simulink model "SoftRoboticTentacle"  (R2024b)
settings: Solver=FixedStepAuto  StartTime=0.0  StopTime=0.1  FixedStep=0.01  RelTol=1e-3
undefined symbols (not defined in the file): c, k, m
settings Model: Creator=Robin  LastModifiedBy=Robin
settings RTWCC: GPUComputeCapability=3.5

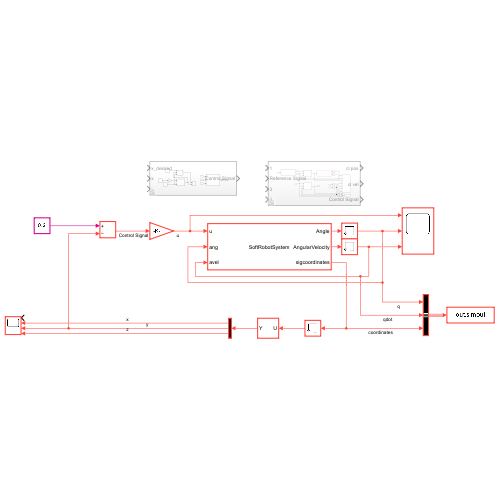
[thumbnail: Simulink's stored preview of the top-level diagram]
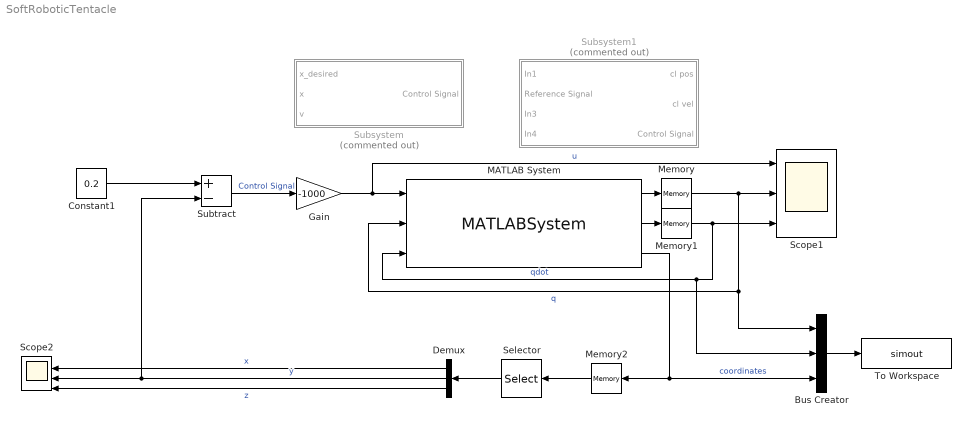
== system SoftRoboticTentacle ==
  Bus Creator : BusCreator  Inputs=3
  Constant1 : Constant  Value=0.2
  Demux : Demux  Outputs=3
  Gain : Gain  Gain=-1000
  MATLAB System : MATLABSystem  System=SoftRobotSystem  SimulateUsing=Interpreted execution
      mask Type: SoftRobotSystem
      mask Display:
      | disp('SoftRobotSystem');
      | port_label('input',1,'u');
      | port_label('input',2,'ang');
      | port_label('input',3,'avel');
      | port_label('output',1,'Angle');
      | port_label('output',2,'AngularVelocity');
      | port_label('output',3,'sigcoordinates');
  Memory : Memory
  Memory1 : Memory
  Memory2 : Memory
  Scope1 : Scope  NumInputPorts=3
  Scope2 : Scope  NumInputPorts=4
  Selector : Selector  InputPortWidth=24  IndexOptions=Index vector (dialog)  Indices=[22 23 24]  OutputSizes=1
  Subsystem : Subsystem  Commented=on
  Subsystem1 : Subsystem  Commented=on
  Subtract : Sum  Inputs=+-
  To Workspace : ToWorkspace  VariableName=simout  SaveFormat=Timeseries  SampleTime=-1
  wires:
  MATLAB System/2 -> Memory1/1
  Bus Creator/1 -> To Workspace/1
  Memory/1 -> Scope1/2, Bus Creator/1, MATLAB System/2  "q"
  Memory1/1 -> Scope1/3, Bus Creator/2, MATLAB System/3  "qdot"
  MATLAB System/1 -> Memory/1
  MATLAB System/3 -> Memory2/1, Bus Creator/3  "coordinates"
  Selector/1 -> Demux/1
  Demux/2 -> Subtract/2, Scope2/3  "y"
  Demux/1 -> Scope2/2  "x"
  Demux/3 -> Scope2/4  "z"
  Constant1/1 -> Subtract/1
  Subtract/1 -> Gain/1  "Control Signal"
  Gain/1 -> Scope1/1, MATLAB System/1  "u"
  Memory2/1 -> Selector/1

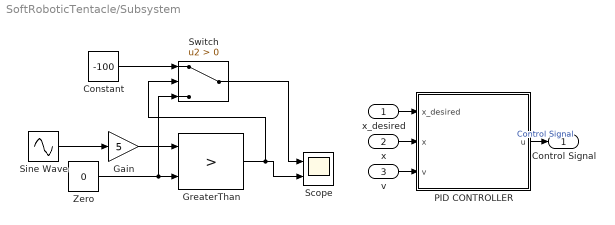
== system SoftRoboticTentacle/Subsystem ==
  x_desired : Inport
  x : Inport  Port=2
  v : Inport  Port=3
  Constant : Constant  Value=-100
  Gain : Gain  Gain=5
  GreaterThan : RelationalOperator  Operator=>  OutDataTypeStr=boolean  RndMeth=Simplest  InputSameDT=off
  PID CONTROLLER : MATLAB Function  TreatAsAtomicUnit=on
  Scope : Scope  NumInputPorts=2
  Sine Wave : Sin  Frequency=10  SampleTime=0
  Switch : Switch  Criteria=u2 > Threshold  SaturateOnIntegerOverflow=off  InputSameDT=off
  Zero : Constant  Value=0  OutDataTypeStr=Inherit: Inherit via back propagation
  Control Signal : Outport
  wires:
  Gain/1 -> GreaterThan/1
  Switch/1 -> Scope/1
  GreaterThan/1 -> Switch/2, Scope/2
  Zero/1 -> Switch/3, GreaterThan/2
  Sine Wave/1 -> Gain/1
  Constant/1 -> Switch/1
  x/1 -> PID CONTROLLER/2(x)
  v/1 -> PID CONTROLLER/3(v)
  x_desired/1 -> PID CONTROLLER/1(x_desired)
  PID CONTROLLER/1(u) -> Control Signal/1  "Control Signal"

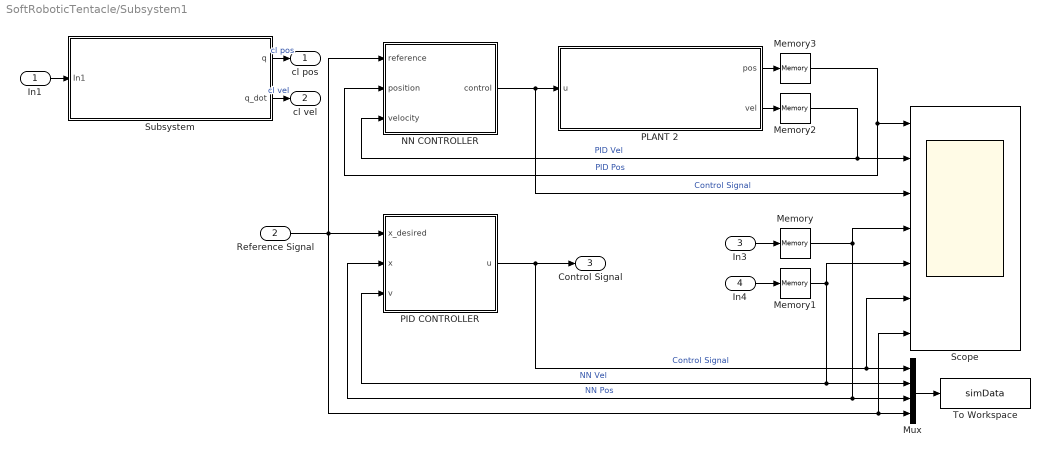
== system SoftRoboticTentacle/Subsystem1 ==
  In1 : Inport
  Reference Signal : Inport  Port=2
  In3 : Inport  Port=3
  In4 : Inport  Port=4
  Memory{,1..3} (4 alike) : Memory
  Mux : Mux
  NN CONTROLLER : MATLAB Function  TreatAsAtomicUnit=on
  PID CONTROLLER : MATLAB Function  TreatAsAtomicUnit=on
  PLANT 2 : MATLAB Function  TreatAsAtomicUnit=on  SystemSampleTime=0.01
  Scope : Scope  NumInputPorts=7
  Subsystem : Subsystem
  To Workspace : ToWorkspace  VariableName=simData  SaveFormat=Structure With Time  SampleTime=-1
  cl pos : Outport
  cl vel : Outport  Port=2
  Control Signal : Outport  Port=3
  wires:
  Memory2/1 -> NN CONTROLLER/3(velocity), Scope/2  "PID Vel"
  Memory/1 -> Scope/4, PID CONTROLLER/2(x), Mux/3  "NN Pos"
  PLANT 2/1(pos) -> Memory3/1
  Memory1/1 -> Scope/5, PID CONTROLLER/3(v), Mux/2  "NN Vel"
  Mux/1 -> To Workspace/1
  PID CONTROLLER/1(u) -> Control Signal/1, Mux/1, Scope/6  "Control Signal"
  NN CONTROLLER/1(control) -> Scope/3, PLANT 2/1(u)  "Control Signal"
  Reference Signal/1 -> PID CONTROLLER/1(x_desired), NN CONTROLLER/1(reference), Scope/7, Mux/4
  Memory3/1 -> NN CONTROLLER/2(position), Scope/1  "PID Pos"
  PLANT 2/2(vel) -> Memory2/1
  In1/1 -> Subsystem/1(In1)
  Subsystem/1(q) -> cl pos/1  "cl pos"
  Subsystem/2(q_dot) -> cl vel/1  "cl vel"
  In4/1 -> Memory1/1
  In3/1 -> Memory/1

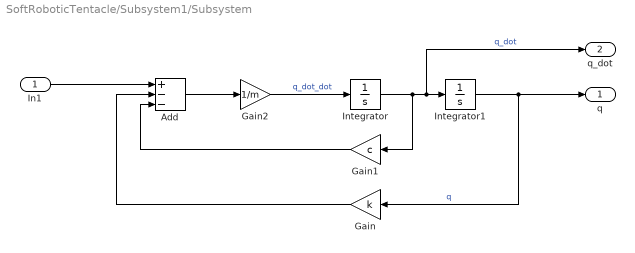
== system SoftRoboticTentacle/Subsystem1/Subsystem ==
  In1 : Inport
  Add : Sum  Inputs=+--
  Gain : Gain  Gain=k
  Gain1 : Gain  Gain=c
  Gain2 : Gain  Gain=1/m
  Integrator : Integrator
  Integrator1 : Integrator
  q : Outport
  q_dot : Outport  Port=2
  wires:
  Gain/1 -> Add/2
  Gain2/1 -> Integrator/1  "q_dot_dot"
  Integrator1/1 -> q/1, Gain/1  "q"
  Gain1/1 -> Add/3
  Integrator/1 -> Gain1/1, q_dot/1, Integrator1/1  "q_dot"
  Add/1 -> Gain2/1
  In1/1 -> Add/1

== matlab function SoftRoboticTentacle/Subsystem1/PID CONTROLLER ==
  settings: updateMethod=DISCRETE
  data: x_desired input; u output; x input; v input
function u = PIDController(x_desired, x, v)
% PIDController - Classic PID controller for mass-spring-damper system
%
% Inputs:
%   x_desired - Desired position (reference)
%   x         - Current position
%   v         - Current velocity
%
% Output:
%   u         - Control force

% Controller gains
Kp = 10;
Ki = 2;
Kd = 2;

% Sample time
Ts = 0.01;

% Persistent PID states
persistent integral_error prev_error
if isempty(integral_error)
    integral_error = 0;
    prev_error = 0;
end

% Compute errors
position_error = x_desired - x;
integral_error = integral_error + position_error * Ts;
derivative_error = (position_error - prev_error) / Ts;

% PID control law
u = Kp * position_error + Ki * integral_error + Kd * derivative_error;

% Optional: Saturation
% u = max(min(u, 10), -10);

% Update persistent state
prev_error = position_error;
end

== matlab function SoftRoboticTentacle/Subsystem/PID CONTROLLER ==
  settings: updateMethod=DISCRETE
  data: x_desired input; u output; x input; v input
function u = PIDController(x_desired, x, v)
% PIDController - Classic PID controller for mass-spring-damper system
%
% Inputs:
%   x_desired - Desired position (reference)
%   x         - Current position
%   v         - Current velocity
%
% Output:
%   u         - Control force

% Controller gains
Kp = 10;
Ki = 2;
Kd = 2;

% Sample time
Ts = 0.01;

% Persistent PID states
persistent integral_error prev_error
if isempty(integral_error)
    integral_error = 0;
    prev_error = 0;
end

% Compute errors
position_error = x_desired - x;
integral_error = integral_error + position_error * Ts;
derivative_error = (position_error - prev_error) / Ts;

% PID control law
u = Kp * position_error + Ki * integral_error + Kd * derivative_error;

% Optional: Saturation
% u = max(min(u, 10), -10);

% Update persistent state
prev_error = position_error;
end

== matlab function SoftRoboticTentacle/Subsystem1/NN CONTROLLER ==
  data: reference input; control output; position input; velocity input
function control = NN_controller(reference, position, velocity)

input = [reference; position; velocity];

control = NNController(input);

== matlab function SoftRoboticTentacle/Subsystem1/PLANT 2 ==
  data: u input; pos output; vel output
function [pos, vel] = massSpringDamperDynamics(u)
% Discrete-time mass-spring-damper system
% u: input force (N)
% pos: output position (m)
% vel: output velocity (m/s)

% System parameters
m = 1.0;    % Mass (kg)
c = 0.5;    % Damping coefficient (Ns/m)
k = 2.0;    % Spring constant (N/m)
Ts = 0.01;  % Sample time (s)

% Persistent state variables
persistent x_prev v_prev
if isempty(x_prev)
    x_prev = 0; % Initial position
    v_prev = 0; % Initial velocity
end

% Compute acceleration
a = (u - c * v_prev - k * x_prev) / m;

% Update states using Euler integration
v = v_prev + Ts * a;
x = x_prev + Ts * v;

% Update persistent variables
v_prev = v;
x_prev = x;

% Output
pos = x;
vel = v;
end
